simulink model "robotarm_A11_pretrained"  (R2018b)
settings: Solver=FixedStepAuto  StartTime=0.0  StopTime=20  RelTol=1e-3  AbsTol=1e-6
undefined symbols (not defined in the file or in its folder): options
libraries: neural x132, simulink x2
(part 2 of 6)

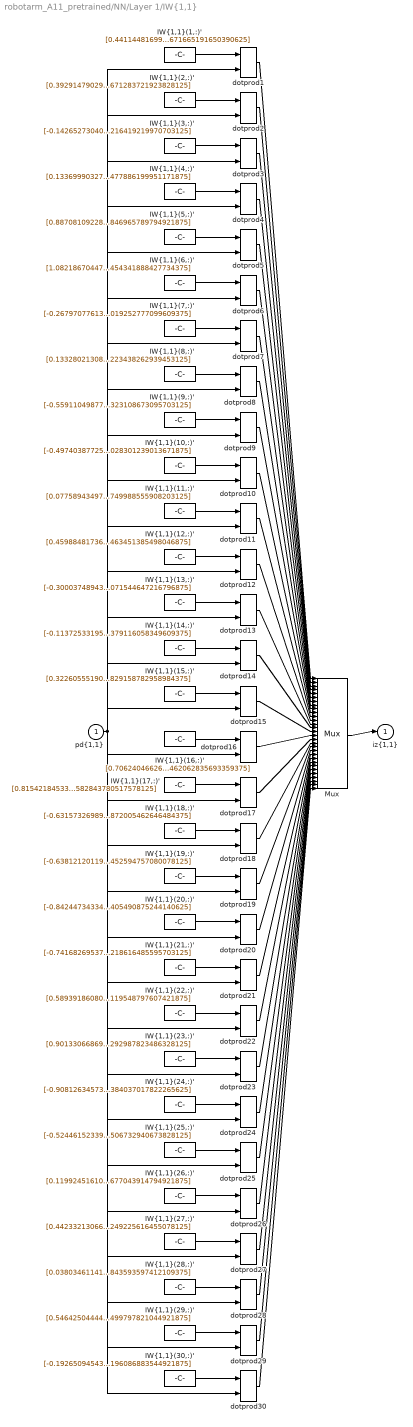
== system robotarm_A11_pretrained/NN/Layer 1/IW{1,1} ==
  "pd{1,1}" : Inport  PortDimensions=10
      mask Display: e = 0.06;c1 = [120 230 180]/255;c2 = ([120 230 180]+0)/(256+128);c3 = ([120 230 180]+128)/(256+128);patch([0 1 1 0],[0 0 1 1],c1);patch([0 1 1 1-e 1-e 0+e],[0 0 1 1-e 0+e 0+e],c2);patch([0 0 1 1-e 0+e 0+e],[0 1 1 1-e 1-e 0+e],c3);plot([0 1 1 0 0],[0 0 1 1 0]);
  "IW{1,1}(1,:)'" : Constant  Value=[0.44114481699030150263496352636138908565044403076171875;0.47057561994338226174505734888953156769275665283203125;-0.161045945358430753202583218808285892009735107421875;0.68876033355921517653541741310618817806243896484375;-0.49145470263358947970999679455417208373546600341796875;0.89641249131439726394177114343619905412197113037109375;-0.6573739199131412025423060185858048498630523681640625;0.037031938519582217883563401983337826095521450042724609375;-0.5783107513623735318475382882752455770969390869140625;0.065251639562963925644822893445962108671665191650390625]
      mask Display: e = 0.06;c1 = [120 150 230]/255;c2 = ([120 150 230]+0)/383;c3 = ([120 150 230]+128)/383;patch([0 1 1 0],[0 0 1 1],c1);patch([0 1 1 1-e 1-e 0+e],[0 0 1 1-e 0+e 0+e],c2);patch([0 0 1 1-e 0+e 0+e],[0 1 1 1-e 1-e 0+e],c3);plot([0 1 1 0 0],[0 0 1 1 0]);disp('Weights');
  "IW{1,1}(10,:)'" : Constant  Value=[-0.49740387725691748155298910205601714551448822021484375;-0.730556425769664397051883497624658048152923583984375;-0.53741187107570720371541028725914657115936279296875;1.109671686326198614125360109028406441211700439453125;-0.466710266010381735757306387313292361795902252197265625;-0.1951083680499688111087408515231800265610218048095703125;0.294283802493082669027302245012833736836910247802734375;0.3341972503424439633334941390785388648509979248046875;0.413880666664230789653089459534385241568088531494140625;0.64446015320846583573910493214498274028301239013671875]
      mask Display: e = 0.06;c1 = [120 150 230]/255;c2 = ([120 150 230]+0)/383;c3 = ([120 150 230]+128)/383;patch([0 1 1 0],[0 0 1 1],c1);patch([0 1 1 1-e 1-e 0+e],[0 0 1 1-e 0+e 0+e],c2);patch([0 0 1 1-e 0+e 0+e],[0 1 1 1-e 1-e 0+e],c3);plot([0 1 1 0 0],[0 0 1 1 0]);disp('Weights');
  "IW{1,1}(11,:)'" : Constant  Value=[0.07758943497745134088017238127577002160251140594482421875;1.1230652360676653955806614249013364315032958984375;-0.73848306599774338199182466269121505320072174072265625;-0.1557297160936446933643395595936453901231288909912109375;0.56574611801836283131450500150094740092754364013671875;-0.6487191398612754955621539920684881508350372314453125;0.41313093161096625660633208099170587956905364990234375;-0.4741330371057286274805164794088341295719146728515625;0.34359999637191507293465519978781230747699737548828125;0.60144024398067597036998677140218205749988555908203125]
      mask Display: e = 0.06;c1 = [120 150 230]/255;c2 = ([120 150 230]+0)/383;c3 = ([120 150 230]+128)/383;patch([0 1 1 0],[0 0 1 1],c1);patch([0 1 1 1-e 1-e 0+e],[0 0 1 1-e 0+e 0+e],c2);patch([0 0 1 1-e 0+e 0+e],[0 1 1 1-e 1-e 0+e],c3);plot([0 1 1 0 0],[0 0 1 1 0]);disp('Weights');
  "IW{1,1}(12,:)'" : Constant  Value=[0.459884817368434284379219434413244016468524932861328125;-0.44196134638367345903731120415613986551761627197265625;0.49308390630628284867498223320581018924713134765625;0.1577530063470549970272571727036847732961177825927734375;-0.69796611588322277075491228970349766314029693603515625;0.77318568598000003699866056194878183305263519287109375;-0.212899809727546351911797728462261147797107696533203125;-0.475708036104746490035921624439652077853679656982421875;0.0753357556053204369117537453348631970584392547607421875;0.69931491253816513431473822492989711463451385498046875]
      mask Display: e = 0.06;c1 = [120 150 230]/255;c2 = ([120 150 230]+0)/383;c3 = ([120 150 230]+128)/383;patch([0 1 1 0],[0 0 1 1],c1);patch([0 1 1 1-e 1-e 0+e],[0 0 1 1-e 0+e 0+e],c2);patch([0 0 1 1-e 0+e 0+e],[0 1 1 1-e 1-e 0+e],c3);plot([0 1 1 0 0],[0 0 1 1 0]);disp('Weights');
  "IW{1,1}(13,:)'" : Constant  Value=[-0.30003748943909547275410432121134363114833831787109375;0.2263079370139092494351729101254022680222988128662109375;0.483534845948699387729874388242023997008800506591796875;-0.411024630408103386347562491209828294813632965087890625;0.15496619406183576028723791750962845981121063232421875;-0.2439842239167192283755269954781397245824337005615234375;-1.1207006345415033710111174514167942106723785400390625;-0.5914188378032012582963261593249626457691192626953125;0.8289392567013340595849513192661106586456298828125;-0.253353668430953138379635447563487105071544647216796875]
      mask Display: e = 0.06;c1 = [120 150 230]/255;c2 = ([120 150 230]+0)/383;c3 = ([120 150 230]+128)/383;patch([0 1 1 0],[0 0 1 1],c1);patch([0 1 1 1-e 1-e 0+e],[0 0 1 1-e 0+e 0+e],c2);patch([0 0 1 1-e 0+e 0+e],[0 1 1 1-e 1-e 0+e],c3);plot([0 1 1 0 0],[0 0 1 1 0]);disp('Weights');
  "IW{1,1}(14,:)'" : Constant  Value=[-0.11372533195621260804220042928136535920202732086181640625;-0.1327798834327793275900120306687313131988048553466796875;0.71745093462888742674721243020030669867992401123046875;-0.55562728456340038096783473520190455019474029541015625;-0.54122733516121623864592038444243371486663818359375;0.7550239742809570220316572886076755821704864501953125;0.68679560816160123426499239940312691032886505126953125;-0.84664501113969581336249348169076256453990936279296875;0.06977763743654173678176988460108987055718898773193359375;-0.43154751694678628037848966414458118379116058349609375]
      mask Display: e = 0.06;c1 = [120 150 230]/255;c2 = ([120 150 230]+0)/383;c3 = ([120 150 230]+128)/383;patch([0 1 1 0],[0 0 1 1],c1);patch([0 1 1 1-e 1-e 0+e],[0 0 1 1-e 0+e 0+e],c2);patch([0 0 1 1-e 0+e 0+e],[0 1 1 1-e 1-e 0+e],c3);plot([0 1 1 0 0],[0 0 1 1 0]);disp('Weights');
  "IW{1,1}(15,:)'" : Constant  Value=[0.322605551906437415521367029214161448180675506591796875;-0.278492656375721014949675691241282038390636444091796875;-0.64538799147380399023887775911134667694568634033203125;0.455871650501271485911303216198575682938098907470703125;0.495248713123296824267782767492462880909442901611328125;-0.930323855192265458668998689972795546054840087890625;0.82195823753056662663851739125675521790981292724609375;-0.42976961283223358289973248247406445443630218505859375;-0.45991562947593944699065104941837489604949951171875;-0.62965017260759681416715238810866139829158782958984375]
      mask Display: e = 0.06;c1 = [120 150 230]/255;c2 = ([120 150 230]+0)/383;c3 = ([120 150 230]+128)/383;patch([0 1 1 0],[0 0 1 1],c1);patch([0 1 1 1-e 1-e 0+e],[0 0 1 1-e 0+e 0+e],c2);patch([0 0 1 1-e 0+e 0+e],[0 1 1 1-e 1-e 0+e],c3);plot([0 1 1 0 0],[0 0 1 1 0]);disp('Weights');
  "IW{1,1}(16,:)'" : Constant  Value=[0.706240466269596023352050906396470963954925537109375;-0.213041370568238297433794059543288312852382659912109375;0.10412508762046095156517111490757088176906108856201171875;0.2386677071228649194001292244138312526047229766845703125;-0.8211409063128589647106991833425126969814300537109375;1.0183460499504992657904267616686411201953887939453125;0.374038038219429658237658031794126145541667938232421875;-0.6265926623906670211994196506566368043422698974609375;-0.729280110188397667769777399371378123760223388671875;-0.341782494837113259844585400060168467462062835693359375]
      mask Display: e = 0.06;c1 = [120 150 230]/255;c2 = ([120 150 230]+0)/383;c3 = ([120 150 230]+128)/383;patch([0 1 1 0],[0 0 1 1],c1);patch([0 1 1 1-e 1-e 0+e],[0 0 1 1-e 0+e 0+e],c2);patch([0 0 1 1-e 0+e 0+e],[0 1 1 1-e 1-e 0+e],c3);plot([0 1 1 0 0],[0 0 1 1 0]);disp('Weights');
  "IW{1,1}(17,:)'" : Constant  Value=[0.8154218453375310371455952918040566146373748779296875;0.73657749410323603012074045182089321315288543701171875;-0.83911559828697412921627574178273789584636688232421875;-0.322821332652742210012064560942235402762889862060546875;0.308925831831681263484057353707612492144107818603515625;-0.59237068710226747914049383325618691742420196533203125;-0.61504641500747470050924903262057341635227203369140625;0.81231889133067924912978696738719008862972259521484375;0.442859438938178084921304389354190789163112640380859375;-0.06637140509416968037204043184829060919582843780517578125]
      mask Display: e = 0.06;c1 = [120 150 230]/255;c2 = ([120 150 230]+0)/383;c3 = ([120 150 230]+128)/383;patch([0 1 1 0],[0 0 1 1],c1);patch([0 1 1 1-e 1-e 0+e],[0 0 1 1-e 0+e 0+e],c2);patch([0 0 1 1-e 0+e 0+e],[0 1 1 1-e 1-e 0+e],c3);plot([0 1 1 0 0],[0 0 1 1 0]);disp('Weights');
  "IW{1,1}(18,:)'" : Constant  Value=[-0.63157326989174211728794716691481880843639373779296875;-0.4161408251964153759416831235284917056560516357421875;0.07940115633735568556605954881888465024530887603759765625;-0.41327102841808838196158149003167636692523956298828125;-0.07312324705246921185963770994931110180914402008056640625;0.2363519030620057914671150456342729739844799041748046875;0.67171041176668655481307723675854504108428955078125;-0.161415698011547370516183264044229872524738311767578125;0.0157607601178772205319233989939675666391849517822265625;-0.494354720976003692012312740189372561872005462646484375]
      mask Display: e = 0.06;c1 = [120 150 230]/255;c2 = ([120 150 230]+0)/383;c3 = ([120 150 230]+128)/383;patch([0 1 1 0],[0 0 1 1],c1);patch([0 1 1 1-e 1-e 0+e],[0 0 1 1-e 0+e 0+e],c2);patch([0 0 1 1-e 0+e 0+e],[0 1 1 1-e 1-e 0+e],c3);plot([0 1 1 0 0],[0 0 1 1 0]);disp('Weights');
  "IW{1,1}(19,:)'" : Constant  Value=[-0.63812120119707260723629360654740594327449798583984375;-0.449120692520197206665244493706268258392810821533203125;0.0252755603751772806031539175819489173591136932373046875;0.031775930868162695352996394149158732034265995025634765625;-0.55120334061858267116207343860878609120845794677734375;0.70803464883989508660278033858048729598522186279296875;0.290034008068234150368169821376795880496501922607421875;-0.2049795497319956416593100811951444484293460845947265625;1.0583939499319405808108740529860369861125946044921875;0.54021326163231286887622673020814545452594757080078125]
      mask Display: e = 0.06;c1 = [120 150 230]/255;c2 = ([120 150 230]+0)/383;c3 = ([120 150 230]+128)/383;patch([0 1 1 0],[0 0 1 1],c1);patch([0 1 1 1-e 1-e 0+e],[0 0 1 1-e 0+e 0+e],c2);patch([0 0 1 1-e 0+e 0+e],[0 1 1 1-e 1-e 0+e],c3);plot([0 1 1 0 0],[0 0 1 1 0]);disp('Weights');
  "IW{1,1}(2,:)'" : Constant  Value=[0.392914790299492999725572417446528561413288116455078125;-0.223438352036276099976674913705210201442241668701171875;-0.91317289066929763219349069913732819259166717529296875;-0.57202707780105932489078668368165381252765655517578125;1.004683557933450099852734638261608779430389404296875;-0.1705981898507127614283973571218666620552539825439453125;-0.27710380432584980070487290504388511180877685546875;0.377845507227642485315044496019254438579082489013671875;-0.8799456694779674847950445837341248989105224609375;0.155434465293079526748698526716907508671283721923828125]
      mask Display: e = 0.06;c1 = [120 150 230]/255;c2 = ([120 150 230]+0)/383;c3 = ([120 150 230]+128)/383;patch([0 1 1 0],[0 0 1 1],c1);patch([0 1 1 1-e 1-e 0+e],[0 0 1 1-e 0+e 0+e],c2);patch([0 0 1 1-e 0+e 0+e],[0 1 1 1-e 1-e 0+e],c3);plot([0 1 1 0 0],[0 0 1 1 0]);disp('Weights');
  "IW{1,1}(20,:)'" : Constant  Value=[-0.84244734334086379679007450249628163874149322509765625;-0.52228267177522214037566072875051759183406829833984375;0.5655555970384400499284538454958237707614898681640625;0.82247803732519508823628484606160782277584075927734375;0.62851041112361638596439661341719329357147216796875;-0.0117758191394388041228769026247391593642532825469970703125;0.036654480047115078900077378420974127948284149169921875;-0.41004048468668397031677841368946246802806854248046875;-0.356003304414170107516923735602176748216152191162109375;-0.46895342613768564721254961114027537405490875244140625]
      mask Display: e = 0.06;c1 = [120 150 230]/255;c2 = ([120 150 230]+0)/383;c3 = ([120 150 230]+128)/383;patch([0 1 1 0],[0 0 1 1],c1);patch([0 1 1 1-e 1-e 0+e],[0 0 1 1-e 0+e 0+e],c2);patch([0 0 1 1-e 0+e 0+e],[0 1 1 1-e 1-e 0+e],c3);plot([0 1 1 0 0],[0 0 1 1 0]);disp('Weights');
  "IW{1,1}(21,:)'" : Constant  Value=[-0.74168269537759012877131681307218968868255615234375;1.40730496612774569342718677944503724575042724609375;-0.5435265139305567316796441446058452129364013671875;0.340510427675548843495789697044529020786285400390625;0.1386778331726278568059029794312664307653903961181640625;-0.8490590474083543615080316158127970993518829345703125;0.30936965875740540798943811751087196171283721923828125;0.09247476949920900579638072258603642694652080535888671875;-0.1782232344620747477303979167118086479604244232177734375;-0.196652854681414357429503070306964218616485595703125]
      mask Display: e = 0.06;c1 = [120 150 230]/255;c2 = ([120 150 230]+0)/383;c3 = ([120 150 230]+128)/383;patch([0 1 1 0],[0 0 1 1],c1);patch([0 1 1 1-e 1-e 0+e],[0 0 1 1-e 0+e 0+e],c2);patch([0 0 1 1-e 0+e 0+e],[0 1 1 1-e 1-e 0+e],c3);plot([0 1 1 0 0],[0 0 1 1 0]);disp('Weights');
  "IW{1,1}(22,:)'" : Constant  Value=[0.5893918608039248052676839506602846086025238037109375;0.79379480725777395999642749302438460290431976318359375;0.472655158404600428401209910589386709034442901611328125;-0.3730101470957973841535704195848666131496429443359375;0.293542406419969592601404428933165036141872406005859375;0.73923332174289624330043579902849160134792327880859375;-0.038635998804612277368608630467861075885593891143798828125;-0.216662657450471252129631238858564756810665130615234375;0.7743168124059074397536051037604920566082000732421875;-0.856216023470505405157382483594119548797607421875]
      mask Display: e = 0.06;c1 = [120 150 230]/255;c2 = ([120 150 230]+0)/383;c3 = ([120 150 230]+128)/383;patch([0 1 1 0],[0 0 1 1],c1);patch([0 1 1 1-e 1-e 0+e],[0 0 1 1-e 0+e 0+e],c2);patch([0 0 1 1-e 0+e 0+e],[0 1 1 1-e 1-e 0+e],c3);plot([0 1 1 0 0],[0 0 1 1 0]);disp('Weights');
  "IW{1,1}(23,:)'" : Constant  Value=[0.9013306686963236113996345011400990188121795654296875;-0.16883308146231745805465607190853916108608245849609375;0.455877105934794413233390741879702545702457427978515625;-0.6724628747575118747903388793929480016231536865234375;-0.0908697517806775767468252524849958717823028564453125;-0.2386019354049108420756653003991232253611087799072265625;-0.65541442450855014190125302775413729250431060791015625;0.1499767143910053224242773239893722347915172576904296875;-0.76415062568237790419090060822782106697559356689453125;0.2763150685977564524620220254291780292987823486328125]
      mask Display: e = 0.06;c1 = [120 150 230]/255;c2 = ([120 150 230]+0)/383;c3 = ([120 150 230]+128)/383;patch([0 1 1 0],[0 0 1 1],c1);patch([0 1 1 1-e 1-e 0+e],[0 0 1 1-e 0+e 0+e],c2);patch([0 0 1 1-e 0+e 0+e],[0 1 1 1-e 1-e 0+e],c3);plot([0 1 1 0 0],[0 0 1 1 0]);disp('Weights');
  "IW{1,1}(24,:)'" : Constant  Value=[-0.908126345736061768576519170892424881458282470703125;0.2016305690981307907616582042464870028197765350341796875;0.40229063715498003528381332216667942702770233154296875;-0.3137645514272378033382437934051267802715301513671875;1.36679862213892722166974635911174118518829345703125;-0.28395861664827248826981076490483246743679046630859375;0.1665485578903851127119395414410973899066448211669921875;0.029162527605095404925616975333468872122466564178466796875;-0.2444365181410098342151826500412425957620143890380859375;-0.006023442876772263677997987230128273949958384037017822265625]
      mask Display: e = 0.06;c1 = [120 150 230]/255;c2 = ([120 150 230]+0)/383;c3 = ([120 150 230]+128)/383;patch([0 1 1 0],[0 0 1 1],c1);patch([0 1 1 1-e 1-e 0+e],[0 0 1 1-e 0+e 0+e],c2);patch([0 0 1 1-e 0+e 0+e],[0 1 1 1-e 1-e 0+e],c3);plot([0 1 1 0 0],[0 0 1 1 0]);disp('Weights');
  "IW{1,1}(25,:)'" : Constant  Value=[-0.524461523394273765319439917220734059810638427734375;-0.59214948467958417044343377710902132093906402587890625;0.05043350992857677239644687006148160435259342193603515625;0.75139965993134227861816043514409102499485015869140625;0.42058080145795850857126652044826187193393707275390625;0.87176815112361338844237934608827345073223114013671875;-0.309831264933599026534238873864524066448211669921875;0.7262115815481469116576818123576231300830841064453125;-0.8107506713344723170422412295010872185230255126953125;-0.146793709471356337292746729872305877506732940673828125]
      mask Display: e = 0.06;c1 = [120 150 230]/255;c2 = ([120 150 230]+0)/383;c3 = ([120 150 230]+128)/383;patch([0 1 1 0],[0 0 1 1],c1);patch([0 1 1 1-e 1-e 0+e],[0 0 1 1-e 0+e 0+e],c2);patch([0 0 1 1-e 0+e 0+e],[0 1 1 1-e 1-e 0+e],c3);plot([0 1 1 0 0],[0 0 1 1 0]);disp('Weights');
  "IW{1,1}(26,:)'" : Constant  Value=[0.11992451610155473173957574317682883702218532562255859375;-0.035210547337792434674508257330671767704188823699951171875;0.207299403661930170539307027866016142070293426513671875;0.5105554004391368305704190788674168288707733154296875;0.487491725383969398688321916779386810958385467529296875;0.6104326068535625982036663117469288408756256103515625;0.431569946092005218840625957454903982579708099365234375;0.6075935760282626940664840731187723577022552490234375;-0.7728287427923994368228477469529025256633758544921875;-0.5354256169438549317618480927194468677043914794921875]
      mask Display: e = 0.06;c1 = [120 150 230]/255;c2 = ([120 150 230]+0)/383;c3 = ([120 150 230]+128)/383;patch([0 1 1 0],[0 0 1 1],c1);patch([0 1 1 1-e 1-e 0+e],[0 0 1 1-e 0+e 0+e],c2);patch([0 0 1 1-e 0+e 0+e],[0 1 1 1-e 1-e 0+e],c3);plot([0 1 1 0 0],[0 0 1 1 0]);disp('Weights');
  "IW{1,1}(27,:)'" : Constant  Value=[0.44233213066665066914850967805250547826290130615234375;-0.13730079600140754347847860117326490581035614013671875;-0.317337428064021154217044795586843974888324737548828125;0.764806886782281480918754823505878448486328125;-0.318596404338633065744801342589198611676692962646484375;-0.8957876920590450708914431743323802947998046875;0.91742319877945266437535565273719839751720428466796875;-0.08422092617729055874509214163481374271214008331298828125;0.8446751758897217410293478678795509040355682373046875;-0.373481564753852801619160572954569943249225616455078125]
      mask Display: e = 0.06;c1 = [120 150 230]/255;c2 = ([120 150 230]+0)/383;c3 = ([120 150 230]+128)/383;patch([0 1 1 0],[0 0 1 1],c1);patch([0 1 1 1-e 1-e 0+e],[0 0 1 1-e 0+e 0+e],c2);patch([0 0 1 1-e 0+e 0+e],[0 1 1 1-e 1-e 0+e],c3);plot([0 1 1 0 0],[0 0 1 1 0]);disp('Weights');
  "IW{1,1}(28,:)'" : Constant  Value=[0.038034611419856916014747838516996125690639019012451171875;-0.205977167814045791782717742535169236361980438232421875;0.73121977697043838428925255357171408832073211669921875;-0.212622628864914009483300105785019695758819580078125;0.72722064631157212755141472371178679168224334716796875;-0.55592303298346268380925039309659041464328765869140625;-0.9632704920535510861867578569217585027217864990234375;0.36891338478317037274933909429819323122501373291015625;-1.02343521627568545540043487562797963619232177734375;-0.353713155995795280883697842000401578843593597412109375]
      mask Display: e = 0.06;c1 = [120 150 230]/255;c2 = ([120 150 230]+0)/383;c3 = ([120 150 230]+128)/383;patch([0 1 1 0],[0 0 1 1],c1);patch([0 1 1 1-e 1-e 0+e],[0 0 1 1-e 0+e 0+e],c2);patch([0 0 1 1-e 0+e 0+e],[0 1 1 1-e 1-e 0+e],c3);plot([0 1 1 0 0],[0 0 1 1 0]);disp('Weights');
  "IW{1,1}(29,:)'" : Constant  Value=[0.54642504444925965589874294892069883644580841064453125;0.62170762183957972712988748753559775650501251220703125;-0.428987541220960555410357528671738691627979278564453125;-0.86032309214516466955302576025133021175861358642578125;-0.258040355820329636582499688302050344645977020263671875;-0.788681952095760419041425848263315856456756591796875;-0.7601611462866684210126777543337084352970123291015625;-0.04431170832280761917587597054080106317996978759765625;0.7497649690672008038205831326195038855075836181640625;0.08175712250195736607860652611634577624499797821044921875]
      mask Display: e = 0.06;c1 = [120 150 230]/255;c2 = ([120 150 230]+0)/383;c3 = ([120 150 230]+128)/383;patch([0 1 1 0],[0 0 1 1],c1);patch([0 1 1 1-e 1-e 0+e],[0 0 1 1-e 0+e 0+e],c2);patch([0 0 1 1-e 0+e 0+e],[0 1 1 1-e 1-e 0+e],c3);plot([0 1 1 0 0],[0 0 1 1 0]);disp('Weights');
  "IW{1,1}(3,:)'" : Constant  Value=[-0.142652730409756844931479236038285307586193084716796875;0.770852997124893857261440643924288451671600341796875;-0.59364405874076442426456878820317797362804412841796875;-0.5669069406306761482738920676638372242450714111328125;-0.331846323074446447609631150044151581823825836181640625;-0.001070568560079488036607120449161811848171055316925048828125;-0.57408727863866182428154161243583075702190399169921875;-0.7657901270849312158617294699070043861865997314453125;0.897660140576344023344290690147317945957183837890625;-0.054383742630841232224003789497146499343216419219970703125]
      mask Display: e = 0.06;c1 = [120 150 230]/255;c2 = ([120 150 230]+0)/383;c3 = ([120 150 230]+128)/383;patch([0 1 1 0],[0 0 1 1],c1);patch([0 1 1 1-e 1-e 0+e],[0 0 1 1-e 0+e 0+e],c2);patch([0 0 1 1-e 0+e 0+e],[0 1 1 1-e 1-e 0+e],c3);plot([0 1 1 0 0],[0 0 1 1 0]);disp('Weights');
  "IW{1,1}(30,:)'" : Constant  Value=[-0.192650945437063902954122340815956704318523406982421875;0.1705933538491863077357635347652831114828586578369140625;0.7029736991586350569605201599188148975372314453125;0.052713413334386706454726123638465651310980319976806640625;0.505456029923756933186496098642237484455108642578125;-0.60028068218333718863988224256900139153003692626953125;-1.0685623989584736026614564252668060362339019775390625;0.31400991831967217660093183440039865672588348388671875;-0.7948918273263025913166757163708098232746124267578125;-0.7652460550642679049104799560154788196086883544921875]
      mask Display: e = 0.06;c1 = [120 150 230]/255;c2 = ([120 150 230]+0)/383;c3 = ([120 150 230]+128)/383;patch([0 1 1 0],[0 0 1 1],c1);patch([0 1 1 1-e 1-e 0+e],[0 0 1 1-e 0+e 0+e],c2);patch([0 0 1 1-e 0+e 0+e],[0 1 1 1-e 1-e 0+e],c3);plot([0 1 1 0 0],[0 0 1 1 0]);disp('Weights');
  "IW{1,1}(4,:)'" : Constant  Value=[0.1336999032767158535062179680608096532523632049560546875;0.1701939170159963155004589907548506744205951690673828125;0.420416237259778002854915257557877339422702789306640625;-1.085407844388667886192934020073153078556060791015625;-0.72006502039104003376479568032664246857166290283203125;0.481538855406381360868550700615742243826389312744140625;-0.58105478390426867907336827556719072163105010986328125;-0.439375147322198233990064863974112085998058319091796875;-0.71570491143323045069024601616547442972660064697265625;-0.170656597084133110353576512352447025477886199951171875]
      mask Display: e = 0.06;c1 = [120 150 230]/255;c2 = ([120 150 230]+0)/383;c3 = ([120 150 230]+128)/383;patch([0 1 1 0],[0 0 1 1],c1);patch([0 1 1 1-e 1-e 0+e],[0 0 1 1-e 0+e 0+e],c2);patch([0 0 1 1-e 0+e 0+e],[0 1 1 1-e 1-e 0+e],c3);plot([0 1 1 0 0],[0 0 1 1 0]);disp('Weights');
  "IW{1,1}(5,:)'" : Constant  Value=[0.887081092285922689910648841760121285915374755859375;-0.1283551137183402690578049032410490326583385467529296875;-0.04797130572346298971186939752442413009703159332275390625;-1.248140968169683784338985788053832948207855224609375;-0.494385200178179162744385166661231778562068939208984375;0.5067787677192743256426865627872757613658905029296875;0.212680242211218561987351449715788476169109344482421875;0.22675334324815654696294586756266653537750244140625;-0.3119512452000596791634734472609125077724456787109375;0.85930393042260966307566150135244242846965789794921875]
      mask Display: e = 0.06;c1 = [120 150 230]/255;c2 = ([120 150 230]+0)/383;c3 = ([120 150 230]+128)/383;patch([0 1 1 0],[0 0 1 1],c1);patch([0 1 1 1-e 1-e 0+e],[0 0 1 1-e 0+e 0+e],c2);patch([0 0 1 1-e 0+e 0+e],[0 1 1 1-e 1-e 0+e],c3);plot([0 1 1 0 0],[0 0 1 1 0]);disp('Weights');
  "IW{1,1}(6,:)'" : Constant  Value=[1.0821867044788628930973573005758225917816162109375;-0.052566732217766358459254405488536576740443706512451171875;0.450528276633832824860093069219146855175495147705078125;-1.18044216682641689430965925566852092742919921875;-0.036197983767445728042755348496939404867589473724365234375;-0.489758845158802691432953224648372270166873931884765625;0.2327245908933519291661440320240217261016368865966796875;0.412832515007964584441424449323676526546478271484375;-0.64641614203374342384478268286329694092273712158203125;-0.34079541142838587486352253108634613454341888427734375]
      mask Display: e = 0.06;c1 = [120 150 230]/255;c2 = ([120 150 230]+0)/383;c3 = ([120 150 230]+128)/383;patch([0 1 1 0],[0 0 1 1],c1);patch([0 1 1 1-e 1-e 0+e],[0 0 1 1-e 0+e 0+e],c2);patch([0 0 1 1-e 0+e 0+e],[0 1 1 1-e 1-e 0+e],c3);plot([0 1 1 0 0],[0 0 1 1 0]);disp('Weights');
  "IW{1,1}(7,:)'" : Constant  Value=[-0.267970776134341892582568789293873123824596405029296875;-0.58122068731560572185657065347186289727687835693359375;0.380263930445323750095809600679785944521427154541015625;0.8037074940125368271992556401528418064117431640625;0.54789936286423657207933501922525465488433837890625;-0.6445095122855459823796309137833304703235626220703125;-0.63173120001618221497352578808204270899295806884765625;0.78938888546546781554980043438263237476348876953125;0.9524139341830653027187736370251514017581939697265625;0.07588228234525561111123437285641557537019252777099609375]
      mask Display: e = 0.06;c1 = [120 150 230]/255;c2 = ([120 150 230]+0)/383;c3 = ([120 150 230]+128)/383;patch([0 1 1 0],[0 0 1 1],c1);patch([0 1 1 1-e 1-e 0+e],[0 0 1 1-e 0+e 0+e],c2);patch([0 0 1 1-e 0+e 0+e],[0 1 1 1-e 1-e 0+e],c3);plot([0 1 1 0 0],[0 0 1 1 0]);disp('Weights');
  "IW{1,1}(8,:)'" : Constant  Value=[0.133280213080834875061242428273544646799564361572265625;0.849778521196260516745724089560098946094512939453125;-1.302290464448134788000288608600385487079620361328125;-0.00477222271569044224903688444783256272785365581512451171875;0.68149303276776185267493701758212409913539886474609375;-0.31181921346424890106874272532877512276172637939453125;-0.206632025245694739279400664599961601197719573974609375;0.6908466380023934316767508789780549705028533935546875;-0.224410380514392715500804342809715308248996734619140625;0.60126060926376823090322432108223438262939453125]
      mask Display: e = 0.06;c1 = [120 150 230]/255;c2 = ([120 150 230]+0)/383;c3 = ([120 150 230]+128)/383;patch([0 1 1 0],[0 0 1 1],c1);patch([0 1 1 1-e 1-e 0+e],[0 0 1 1-e 0+e 0+e],c2);patch([0 0 1 1-e 0+e 0+e],[0 1 1 1-e 1-e 0+e],c3);plot([0 1 1 0 0],[0 0 1 1 0]);disp('Weights');
  "IW{1,1}(9,:)'" : Constant  Value=[-0.55911049877604279689791155760758556425571441650390625;-0.15651723719747112628652985222288407385349273681640625;0.68830749835243587586575131354038603603839874267578125;0.495842486638183033154092527183820493519306182861328125;0.53064341472015719158861202231491915881633758544921875;0.7394142460629453683651490791817195713520050048828125;0.54355810729347042720149829619913361966609954833984375;0.2002826537383731453356716656344360671937465667724609375;0.1983608802250813596401712857186794281005859375;0.6034384801557675093164334612083621323108673095703125]
      mask Display: e = 0.06;c1 = [120 150 230]/255;c2 = ([120 150 230]+0)/383;c3 = ([120 150 230]+128)/383;patch([0 1 1 0],[0 0 1 1],c1);patch([0 1 1 1-e 1-e 0+e],[0 0 1 1-e 0+e 0+e],c2);patch([0 0 1 1-e 0+e 0+e],[0 1 1 1-e 1-e 0+e],c3);plot([0 1 1 0 0],[0 0 1 1 0]);disp('Weights');
  Mux : Mux  Inputs=30
      mask Display: e = 0.06;c1 = [120 150 230]/255;c2 = ([120 150 230]+0)/383;c3 = ([120 150 230]+128)/383;patch([0 1 1 0],[0 0 1 1],c1);patch([0 1 1 1-e 1-e 0+e],[0 0 1 1-e 0+e 0+e],c2);patch([0 0 1 1-e 0+e 0+e],[0 1 1 1-e 1-e 0+e],c3);plot([0 1 1 0 0],[0 0 1 1 0]);disp('Mux');
  dotprod{1..30} (30 alike) : neural/Weight Functions/dotprod
  "iz{1,1}" : Outport
      mask Display: e = 0.06;c1 = [120 230 180]/255;c2 = ([120 230 180]+0)/(256+128);c3 = ([120 230 180]+128)/(256+128);patch([0 1 1 0],[0 0 1 1],c1);patch([0 1 1 1-e 1-e 0+e],[0 0 1 1-e 0+e 0+e],c2);patch([0 0 1 1-e 0+e 0+e],[0 1 1 1-e 1-e 0+e],c3);plot([0 1 1 0 0],[0 0 1 1 0]);
  wires:
  "IW{1,1}(1,:)'"/1 -> dotprod1/1
  "pd{1,1}"/1 -> dotprod1/2, dotprod2/2, dotprod3/2, dotprod4/2, dotprod5/2, dotprod6/2, dotprod7/2, dotprod8/2, dotprod9/2, dotprod10/2, dotprod11/2, dotprod12/2, dotprod13/2, dotprod14/2, dotprod15/2, dotprod16/2, dotprod17/2, dotprod18/2, dotprod19/2, dotprod20/2, dotprod21/2, dotprod22/2, dotprod23/2, dotprod24/2, dotprod25/2, dotprod26/2, dotprod27/2, dotprod28/2, dotprod29/2, dotprod30/2
  dotprod1/1 -> Mux/1
  "IW{1,1}(2,:)'"/1 -> dotprod2/1
  dotprod2/1 -> Mux/2
  "IW{1,1}(3,:)'"/1 -> dotprod3/1
  dotprod3/1 -> Mux/3
  "IW{1,1}(4,:)'"/1 -> dotprod4/1
  dotprod4/1 -> Mux/4
  "IW{1,1}(5,:)'"/1 -> dotprod5/1
  dotprod5/1 -> Mux/5
  "IW{1,1}(6,:)'"/1 -> dotprod6/1
  dotprod6/1 -> Mux/6
  "IW{1,1}(7,:)'"/1 -> dotprod7/1
  dotprod7/1 -> Mux/7
  "IW{1,1}(8,:)'"/1 -> dotprod8/1
  dotprod8/1 -> Mux/8
  "IW{1,1}(9,:)'"/1 -> dotprod9/1
  dotprod9/1 -> Mux/9
  "IW{1,1}(10,:)'"/1 -> dotprod10/1
  dotprod10/1 -> Mux/10
  "IW{1,1}(11,:)'"/1 -> dotprod11/1
  dotprod11/1 -> Mux/11
  "IW{1,1}(12,:)'"/1 -> dotprod12/1
  dotprod12/1 -> Mux/12
  "IW{1,1}(13,:)'"/1 -> dotprod13/1
  dotprod13/1 -> Mux/13
  "IW{1,1}(14,:)'"/1 -> dotprod14/1
  dotprod14/1 -> Mux/14
  "IW{1,1}(15,:)'"/1 -> dotprod15/1
  dotprod15/1 -> Mux/15
  "IW{1,1}(16,:)'"/1 -> dotprod16/1
  dotprod16/1 -> Mux/16
  "IW{1,1}(17,:)'"/1 -> dotprod17/1
  dotprod17/1 -> Mux/17
  "IW{1,1}(18,:)'"/1 -> dotprod18/1
  dotprod18/1 -> Mux/18
  "IW{1,1}(19,:)'"/1 -> dotprod19/1
  dotprod19/1 -> Mux/19
  "IW{1,1}(20,:)'"/1 -> dotprod20/1
  dotprod20/1 -> Mux/20
  "IW{1,1}(21,:)'"/1 -> dotprod21/1
  dotprod21/1 -> Mux/21
  "IW{1,1}(22,:)'"/1 -> dotprod22/1
  dotprod22/1 -> Mux/22
  "IW{1,1}(23,:)'"/1 -> dotprod23/1
  dotprod23/1 -> Mux/23
  "IW{1,1}(24,:)'"/1 -> dotprod24/1
  dotprod24/1 -> Mux/24
  "IW{1,1}(25,:)'"/1 -> dotprod25/1
  dotprod25/1 -> Mux/25
  "IW{1,1}(26,:)'"/1 -> dotprod26/1
  dotprod26/1 -> Mux/26
  "IW{1,1}(27,:)'"/1 -> dotprod27/1
  dotprod27/1 -> Mux/27
  "IW{1,1}(28,:)'"/1 -> dotprod28/1
  dotprod28/1 -> Mux/28
  "IW{1,1}(29,:)'"/1 -> dotprod29/1
  dotprod29/1 -> Mux/29
  "IW{1,1}(30,:)'"/1 -> dotprod30/1
  dotprod30/1 -> Mux/30
  Mux/1 -> "iz{1,1}"/1

== system robotarm_A11_pretrained/NN/Layer 2/Delays 1 ==
  "p{2}" : Inport  PortDimensions=30
      mask Display: e = 0.06;c1 = [120 230 180]/255;c2 = ([120 230 180]+0)/(256+128);c3 = ([120 230 180]+128)/(256+128);patch([0 1 1 0],[0 0 1 1],c1);patch([0 1 1 1-e 1-e 0+e],[0 0 1 1-e 0+e 0+e],c2);patch([0 0 1 1-e 0+e 0+e],[0 1 1 1-e 1-e 0+e],c3);plot([0 1 1 0 0],[0 0 1 1 0]);
  mux : Mux  Inputs=1
      mask Display: e = 0.06;c1 = [120 150 230]/255;c2 = ([120 150 230]+0)/383;c3 = ([120 150 230]+128)/383;patch([0 1 1 0],[0 0 1 1],c1);patch([0 1 1 1-e 1-e 0+e],[0 0 1 1-e 0+e 0+e],c2);patch([0 0 1 1-e 0+e 0+e],[0 1 1 1-e 1-e 0+e],c3);plot([0 1 1 0 0],[0 0 1 1 0]);disp('Mux')
  "pd{2,1}" : Outport
      mask Display: e = 0.06;c1 = [120 230 180]/255;c2 = ([120 230 180]+0)/(256+128);c3 = ([120 230 180]+128)/(256+128);patch([0 1 1 0],[0 0 1 1],c1);patch([0 1 1 1-e 1-e 0+e],[0 0 1 1-e 0+e 0+e],c2);patch([0 0 1 1-e 0+e 0+e],[0 1 1 1-e 1-e 0+e],c3);plot([0 1 1 0 0],[0 0 1 1 0]);
  wires:
  "p{2}"/1 -> mux/1
  mux/1 -> "pd{2,1}"/1
